simulink model "zad5"  (R2023b)
settings: Solver=VariableStepAuto  StartTime=0.0  StopTime=30  RelTol=1e-3
settings Model: Creator=mkmac  LastModifiedBy=Lenovo

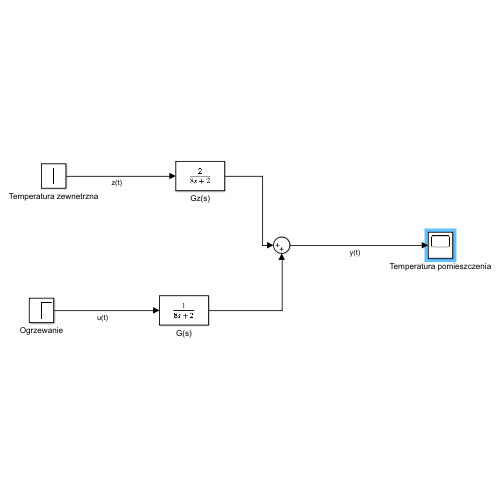
[thumbnail: Simulink's stored preview of the top-level diagram]
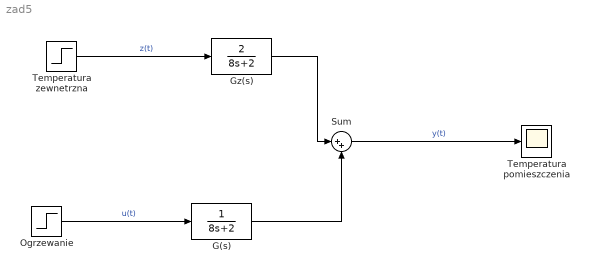
== system zad5 ==
  G(s) : TransferFcn  Denominator=[8 2]
  Gz(s) : TransferFcn  Numerator=[2]  Denominator=[8 2]
  Ogrzewanie : Step  Time=3  SampleTime=0
  Sum : Sum  Inputs=|++
  Temperatura pomieszczenia : Scope
  Temperatura zewnetrzna : Step  Time=2  After=-2  SampleTime=0
  wires:
  Temperatura zewnetrzna/1 -> Gz(s)/1  "z(t)"
  Ogrzewanie/1 -> G(s)/1  "u(t)"
  G(s)/1 -> Sum/2
  Gz(s)/1 -> Sum/1
  Sum/1 -> Temperatura pomieszczenia/1  "y(t)"
